simulink model "BlockDprob2g_nonlin_sat"  (R2017a)
settings: Solver=VariableStepAuto  StartTime=0.0  StopTime=230.0  RelTol=1e-3
values from neighbouring files (symbols this model uses):
  A = [-0.322, 0.052, 0.028, -1.12 , 0.002;       0     , 0    , 1    , -0.001,     0;       -10.6 , 0    , -2.87, 0.46  , -0.65;       6.87  , 0    , -0.04, -0.32 , -0.02;       0     , 0    , 0    , 0     ,   -10 ]    [run_task_2g.m]
  B = [0 0 0 0 10]'    [run_task_2g.m]
  C = [0 0 0 1 0;       0 0 1 0 0;       1 0 0 0 0;       0 1 0 0 0]    [run_task_2g.m]
  D = zeros(4,1)    [run_task_2g.m]
  k_d_phi = f_kd(zp, wp)    [run_task_2g.m]
  k_i_chi = V_g/g * wx^2    [run_task_2g.m]
  k_i_phi = 0    [run_task_2g.m]
  k_p_chi = V_g/g * 2*zx*wx    [run_task_2g.m]
  k_p_phi = -5/3    (= -1.66666666667)    [run_task_2g.m]
libraries: simulink_extras x4
settings Model: Creator=helene  LastModifiedBy=Jens
settings ConfigComp: DVTestSuiteOptimization=CombinedObjectives (Nonlinear Extended)  DVDetectFloatOverflow=off

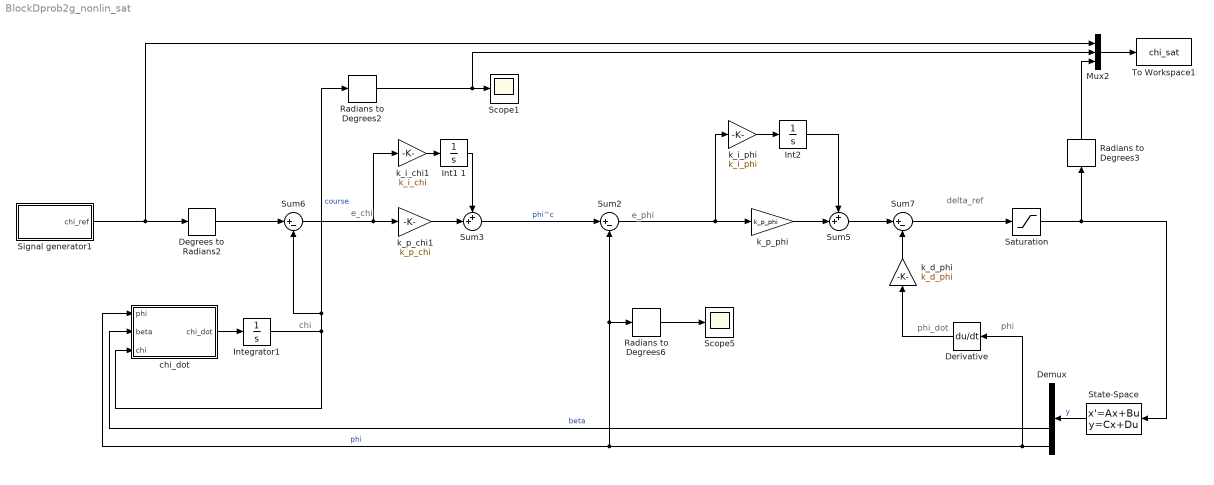
== system BlockDprob2g_nonlin_sat ==
  note: e_chi
  note: chi
  note: phi_dot
  note: e_phi
  note: phi
  note: delta_ref
  Degrees to Radians2 : simulink_extras/Transformations/Degrees to Radians
  Demux : Demux
  Derivative : Derivative
  Int1 1 : Integrator  LimitOutput=on  UpperSaturationLimit=0.15  LowerSaturationLimit=-0.15
  "Int2 " : Integrator
  Integrator1 : Integrator
  Mux2 : Mux  Inputs=3
  Radians to Degrees2 : simulink_extras/Transformations/Radians to Degrees
  Radians to Degrees3 : simulink_extras/Transformations/Radians to Degrees
  Radians to Degrees6 : simulink_extras/Transformations/Radians to Degrees
  Saturation : Saturate  UpperLimit=25*deg2rad  LowerLimit=-25*deg2rad
  Scope1 : Scope
  Scope5 : Scope
  Signal generator1 : Subsystem
  State-Space : StateSpace  A=A  B=B  C=C  D=D  X0=0
  Sum2 : Sum  Inputs=|+-
  Sum3 : Sum  Inputs=++|
  Sum5 : Sum  Inputs=++|
  Sum6 : Sum  Inputs=|+-
  Sum7 : Sum  Inputs=|+-
  To Workspace1 : ToWorkspace  VariableName=chi_sat  SaveFormat=Timeseries  SampleTime=-1
  chi_dot : MATLAB Function  TreatAsAtomicUnit=on
  k_d_phi : Gain  Gain=k_d_phi
  k_i_chi1 : Gain  Gain=k_i_chi
  k_i_phi : Gain  Gain=k_i_phi
  k_p_chi1 : Gain  Gain=k_p_chi
  "k_p_phi " : Gain  Gain=k_p_phi
  wires:
  chi_dot/1(chi_dot) -> Integrator1/1
  k_i_phi/1 -> "Int2 "/1
  "Int2 "/1 -> Sum5/1
  "k_p_phi "/1 -> Sum5/2
  Sum2/1 -> k_i_phi/1, "k_p_phi "/1
  Sum3/1 -> Sum2/1  "phi^c"
  Sum6/1 -> k_i_chi1/1, k_p_chi1/1
  k_p_chi1/1 -> Sum3/2
  k_i_chi1/1 -> Int1 1/1
  Int1 1/1 -> Sum3/1
  Derivative/1 -> k_d_phi/1
  k_d_phi/1 -> Sum7/2
  Degrees to Radians2/1 -> Sum6/1
  Radians to Degrees2/1 -> Mux2/2, Scope1/1
  Radians to Degrees6/1 -> Scope5/1
  Demux/4 -> Derivative/1, Radians to Degrees6/1, Sum2/2, chi_dot/1(phi)  "phi"
  Mux2/1 -> To Workspace1/1
  Integrator1/1 -> chi_dot/3(chi), Radians to Degrees2/1, Sum6/2  "course"
  Sum5/1 -> Sum7/1
  Sum7/1 -> Saturation/1
  Saturation/1 -> State-Space/1, Radians to Degrees3/1
  State-Space/1 -> Demux/1  "y"
  Demux/3 -> chi_dot/2(beta)  "beta"
  Signal generator1/1(chi_ref) -> Mux2/1, Degrees to Radians2/1
  Radians to Degrees3/1 -> Mux2/3

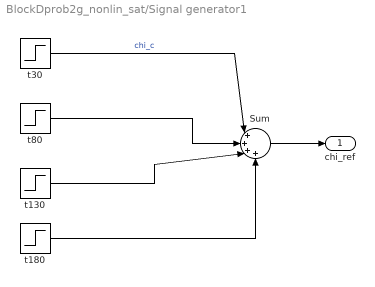
== system BlockDprob2g_nonlin_sat/Signal generator1 ==
  Sum : Sum  Inputs=|++++
  t130 : Step  Time=130  After=-15  SampleTime=0
  t180 : Step  Time=180  After=-10  SampleTime=0
  t30 : Step  Time=30  After=15  SampleTime=0
  "t80 " : Step  Time=80  After=10  SampleTime=0
  chi_ref : Outport
  wires:
  Sum/1 -> chi_ref/1
  t30/1 -> Sum/1  "chi_c"
  "t80 "/1 -> Sum/2
  t130/1 -> Sum/3
  t180/1 -> Sum/4

== matlab function BlockDprob2g_nonlin_sat/chi_dot ==
  data: phi input; beta input; chi input; chi_dot output
function chi_dot = fcn(phi,beta, chi)

d = 2 * pi/180;
g = 9.81; % [m/s^2] gravity
V_g = 637/3.6 ; % [m/s] Speed over ground (637 [km/h]) 

psi  = chi - beta;


chi_dot = g/V_g * tan(phi+d) *cos(chi - psi);
